simulink model "GetBit_SetBit"  (R2016b)
settings: Solver=VariableStepAuto  StartTime=0.0  StopTime=10.0  RelTol=1e-3
libraries: simulink x3
settings Model: Creator=zhoutinglin  LastModifiedBy=zhoutinglin

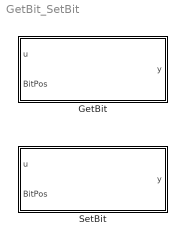
== system GetBit_SetBit ==
  GetBit : Subsystem
      mask DialogControl DescGroupVar Prompt: GetBit
      mask DialogControl DescTextVar Prompt: The two input should has the same Datatype, and can only be one of uint8, uint16 or uint32
  SetBit : Subsystem
      mask DialogControl DescGroupVar Prompt: SetBit
      mask DialogControl DescTextVar Prompt: The two input should has the same Datatype, and can only be one of uint8, uint16 or uint32

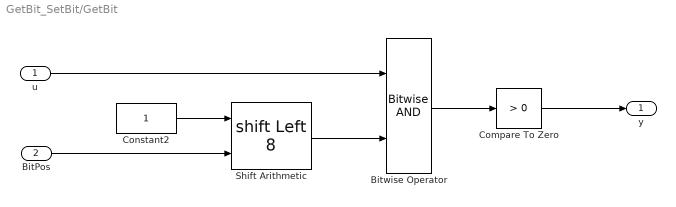
== system GetBit_SetBit/GetBit ==
  u : Inport
  BitPos : Inport  Port=2
  Bitwise Operator : simulink/Logic and Bit Operations/Bitwise Operator  logicop=AND  UseBitMask=off  NumInputPorts=2  BitMask=bin2dec('11011001')  BitMaskRealWorld=Stored Integer
  Compare To Zero : simulink/Logic and Bit Operations/Compare To Zero  relop=>  OutDataTypeStr=boolean  ZeroCross=off
  Constant2 : Constant  OutDataTypeStr=Inherit: Inherit via back propagation
  Shift Arithmetic : ArithShift  BitShiftNumberSource=Input port  BitShiftNumber=8  BitShiftDirection=Left
      settings: InputPortMap=u0,p1
  y : Outport
  wires:
  Compare To Zero/1 -> y/1
  u/1 -> Bitwise Operator/1
  Constant2/1 -> Shift Arithmetic/1
  Shift Arithmetic/1 -> Bitwise Operator/2
  Bitwise Operator/1 -> Compare To Zero/1
  BitPos/1 -> Shift Arithmetic/2

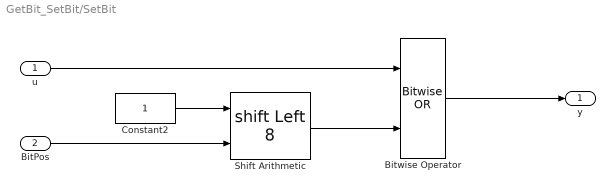
== system GetBit_SetBit/SetBit ==
  u : Inport
  BitPos : Inport  Port=2
  Bitwise Operator : simulink/Logic and Bit Operations/Bitwise Operator  logicop=OR  UseBitMask=off  NumInputPorts=2  BitMask=bin2dec('11011001')  BitMaskRealWorld=Stored Integer
  Constant2 : Constant  OutDataTypeStr=Inherit: Inherit via back propagation
  Shift Arithmetic : ArithShift  BitShiftNumberSource=Input port  BitShiftNumber=8  BitShiftDirection=Left
      settings: InputPortMap=u0,p1
  y : Outport
  wires:
  BitPos/1 -> Shift Arithmetic/2
  Shift Arithmetic/1 -> Bitwise Operator/2
  Constant2/1 -> Shift Arithmetic/1
  u/1 -> Bitwise Operator/1
  Bitwise Operator/1 -> y/1
